simulink model "exp2_3_2_C"  (R2014a)
settings: Solver=ode5  StartTime=0.0  StopTime=inf  RelTol=1e-3
libraries: xpcdiamondlib x2, slrtlib x2
settings Model: BufferReuse=off  Creator=wwang195  LastModifiedBy=dallen6
settings SolverCC: EnableConcurrentExecution=on
settings OptimizationCC: BlockReduction=off  OptimizeBlockIOStorage=off  BufferReuse=off  GlobalBufferReuse=off  ExpressionFolding=off  LocalBlockOutputs=off
settings HardwareCC: ProdIntDivRoundTo=Zero  ProdEndianess=LittleEndian  ProdHWDeviceType=Generic->32-bit x86 compatible
settings RTWCC: SystemTargetFile=slrt.tlc  TemplateMakefile=slrt_default_tmf  Description=Simulink Real-Time  ProcessScript=slrt_make_rtw_hook  RTWCompilerOptimization=On
settings SimulinkRealTimeCC: GeneratePreprocessorConditionals=Disable all  EnableShiftOperators=on

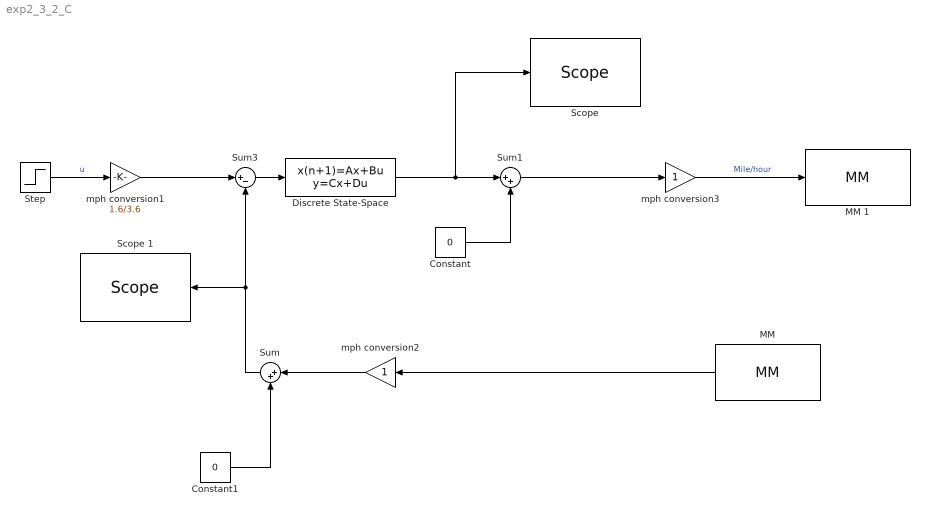
== system exp2_3_2_C ==
  Constant : Constant  Value=0
  Constant1 : Constant  Value=0
  Discrete State-Space : DiscreteStateSpace  B=0.01  C=0.9094  D=1.15  X0=.2606  SampleTime=0.01
  "MM " : xpcdiamondlib/A//D/MM   numChans=1  range=-5V to 5V  coupling=16 single-ended channels  showStatus=off  sampleTime=0.01  base=0x300
  MM 1 : xpcdiamondlib/D//A/MM   channel=[1]  range=[5]  reset=[1]  initValue=[0]  sampleTime=0.01  base=0x300
  "Scope " : slrtlib/Displays and Logging/Scope   scopeno=1  scopetype=File  autostart=on  viewmode=Graphical redraw  formatstr='%15.6f'  grid=on  ylimits=[0,0]  nosamples=5000  noprepostsamples=0  interleave=1  triggermode=FreeRun  triggersignal=1  trigsignalfromport=off  triggerlevel=0.0  triggerslope=Either  triggerscope=1  triggersample=0  filename=data.dat  mode=Lazy  writesize=512  autorestart=on  dynamicfilemode=off  maxwritefilesize=512*1024^2
  Scope 1 : slrtlib/Displays and Logging/Scope   scopeno=2  scopetype=File  autostart=on  viewmode=Graphical redraw  formatstr='%15.6f'  grid=on  ylimits=[0,0]  nosamples=5000  noprepostsamples=0  interleave=1  triggermode=FreeRun  triggersignal=1  trigsignalfromport=off  triggerlevel=0.0  triggerslope=Either  triggerscope=1  triggersample=0  filename=data2.dat  mode=Lazy  writesize=512  autorestart=on  dynamicfilemode=off  maxwritefilesize=512*1024^2
  Step : Step  Time=10  Before=60  After=65  SampleTime=0
  Sum : Sum  Inputs=|++
  Sum1 : Sum  Inputs=|++
  Sum3 : Sum  Inputs=|+-
  mph conversion1 : Gain  Gain=1.6/3.6  SaturateOnIntegerOverflow=on  OutDataTypeStr=Inherit: Same as input  ParamDataTypeStr=Inherit: Same as input
  mph conversion2 : Gain  SaturateOnIntegerOverflow=on  OutDataTypeStr=Inherit: Same as input  ParamDataTypeStr=Inherit: Same as input
  mph conversion3 : Gain  SaturateOnIntegerOverflow=on  OutDataTypeStr=Inherit: Same as input  ParamDataTypeStr=Inherit: Same as input
  wires:
  Step/1 -> mph conversion1/1  "u"
  mph conversion1/1 -> Sum3/1
  Sum3/1 -> Discrete State-Space/1
  Sum/1 -> Scope 1/1, Sum3/2
  mph conversion2/1 -> Sum/1
  "MM "/1 -> mph conversion2/1
  Constant1/1 -> Sum/2
  Discrete State-Space/1 -> "Scope "/1, Sum1/1
  Sum1/1 -> mph conversion3/1
  mph conversion3/1 -> MM 1/1  "Mile/hour"
  Constant/1 -> Sum1/2
